simulink model "process_frame"  (R2021a)
settings: Solver=VariableStepAuto  StartTime=0.0  StopTime=10.0  RelTol=1e-3
undefined symbols (not defined in the file or in its folder): Rec, SDTV
libraries: visionconversions x3, visionsources x1
settings Model: Creator=Owner  LastModifiedBy=Owner

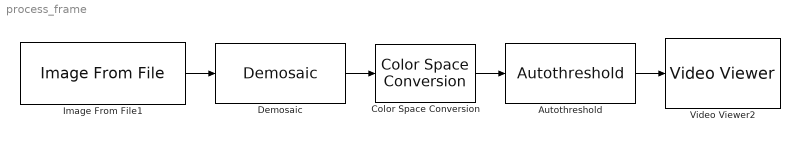
== system process_frame ==
  Autothreshold : visionconversions/Autothreshold  operator=>  threshOut=off  effMetricOut=off  userDefinedRange=off  umin=0  umax=255  outOfRngOpt=Ignore  scaleThreshold=off  scaleFactor=1  roundingMode=Floor  overflowMode=off  P1Mode=Specify word length  P1WordLength=32  P1FracLength=30  P2Mode=Specify word length  P2WordLength=32  P2FracLength=22  P3Mode=Specify word length  P3WordLength=32  P3FracLength=14  P4Mode=Binary point scaling  P4WordLength=32  P4FracLength=15  Q1Mode=Specify word length  Q1WordLength=32  Q1FracLength=16  EMMode=Specify word length  EMWordLength=16  EMFracLength=14
      settings: SourceProductBaseCode=VP
  Color Space Conversion : visionconversions/Color Space  Conversion  conversion=Obsolete  conversionActive=R'G'B' to intensity  wp_str=D65  rec=Rec. 601 (SDTV)  sys=1125/60/2:1  imagePorts=One multidimensional signal
  Demosaic : visionconversions/Demosaic  algorithm=Obsolete  algorithmActive=Bilinear  alignment=RGGB  imagePorts=One multidimensional signal  roundingMode=Floor  overflowMode=on  prodOutputMode=Binary point scaling  prodOutputWordLength=32  prodOutputFracLength=10
      settings: SourceProductBaseCode=VP
  Image From File1 : visionsources/Image From File  Tag=vipblks_nd  FileName=C:\Users\Owner\OneDrive\Documents\Python Scripts\Senior-Design-Project-EMCH427-002-Team-4-Downey\Software\Python\save\video_ai\whole916.png  Ts=inf  imagePorts=One multidimensional signal  OutPortLabels=R|G|B  ImageDataType=Inherit from input image  sdImageDataType=uint(8)  Signed=on  WordLength=16  FractionLengthMode=User-defined  FractionLength=15
  Video Viewer2 : VideoViewer  FigPos=[-499.666666666667 658.666666666667 418 304]
  wires:
  Autothreshold/1 -> Video Viewer2/1
  Color Space Conversion/1 -> Autothreshold/1
  Demosaic/1 -> Color Space Conversion/1
  Image From File1/1 -> Demosaic/1
